simulink model "VU_motorSpdCtrl"  (Simulink 10.0)
settings: Solver=FixedStepDiscrete  StartTime=0.0  StopTime=inf  FixedStep=0.05  RelTol=1e-3  EnableMultiTasking=on
libraries: lego_nxt_lib x2
settings Model: Creator=jpeytonj  LastModifiedBy=bhisma
settings DataIOCC: LimitDataPoints=on  SignalLoggingSaveFormat=ModelDataLogs
settings OptimizationCC: ExpressionDepthLimit=2147483647
settings DebuggingCC: SolverPrmCheckMsg=warning  FcnCallInpInsideContextMsg=warning  StateNameClashWarn=warning
settings SFSimCC: SimParseCustomCode=off
settings RTWCC: Description=Lego NXT Real-Time Target  SystemTargetFile=lrt.tlc  GenCodeOnly=on  TemplateMakefile=lrt_ecrobot.tmf
settings STFCustomTargetCC: ModelReferenceCompliant=off  GeneratePreprocessorConditionals=Disable all  MatFileLogging=on  CPPClassGenCompliant=on  SystemTargetFile=lrt.tlc
settings GRTTargetCC: ModelReferenceCompliant=off  ParMdlRefBuildCompliant=off  CompOptLevelCompliant=off  ConcurrentExecutionCompliant=off  GeneratePreprocessorConditionals=Disable all  UseToolchainInfoCompliant=off  ExtModeMexFile=noextcomm
settings CustomProperty: DataType=RTWOptions_EnumType_C__LegoMindstorms_ECRobot_lrt_lrt_1codeGenType  Value=Integer-only
settings EnumStrPairs: String=Integer-only
settings ConfigComp: CovExternalEMLEnable=off

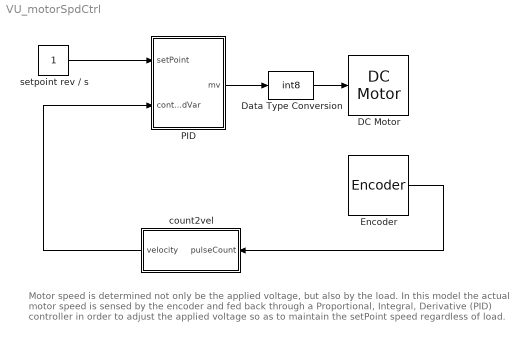
== system VU_motorSpdCtrl ==
  note: Motor speed is determined not only be the applied voltage, but also by the load.
      | In this model the actual motor speed is sensed by the encoder and fed back through
      | a Proportional, Integral, Derivative (PID) controller in order to adjust the applied voltage
      | so as to maintain the setPoint speed regardless of load.
  DC Motor : lego_nxt_lib/DC Motor  port=Port C  brake=Coast
  Data Type Conversion : DataTypeConversion  OutDataTypeStr=int8  SaturateOnIntegerOverflow=on
  Encoder : lego_nxt_lib/Encoder  port=Port C  st=0.05
  PID : Subsystem  mask{Kc=5.5, Ti=1.5, Td=0, mvMax=100, mvMin=-100}
      mask prompts: Kc "Proportional gain:"; Ti "Integral time:"; Td "Derivative time:"; mvMax "Max manipulated output Limit:"; mvMin "Min manipulated output Limit:"
  count2vel : Subsystem  mask(count2vel){gainFactor=1/0.05*1/360}
      mask prompts: gainFactor "Gain Factor:"
      mask help:
      | Use gainFactor to define units of the result:
      | If gainFactor=1, => units of velocity= (pulses/sample).
      | The encoders give 360 pulses / revolution of the output shaft
      |
      | Example:  To obtain velocity in rev/sec
      | velocity = (pulses/sample) * (samples/sec) * (rev/pulses) = rev/sec
      | Given a sample period T=0.1, and the known 360 pulses per rev...
      | => gainFactor = (1/0.1) * (1/360) = 1/36
      |
      | Not clear what happens when the pulse count overflows
  setpoint rev / s : Constant
  wires:
  PID/1(mv) -> Data Type Conversion/1
  setpoint rev / s/1 -> PID/1(setPoint)
  count2vel/1(velocity) -> PID/2(controlledVar)
  Data Type Conversion/1 -> DC Motor/1
  Encoder/1 -> count2vel/1(pulseCount)

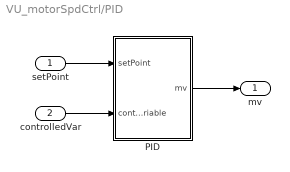
== system VU_motorSpdCtrl/PID ==
  setPoint : Inport
  controlledVar : Inport  Port=2
  PID : MATLAB Function  TreatAsAtomicUnit=on
  mv : Outport
  wires:
  setPoint/1 -> PID/1(setPoint)
  controlledVar/1 -> PID/2(contolledVariable)
  PID/1(mv) -> mv/1

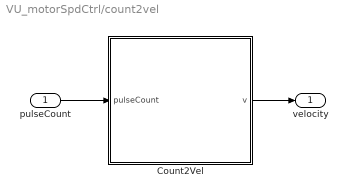
== system VU_motorSpdCtrl/count2vel ==
  pulseCount : Inport
  Count2Vel : MATLAB Function  TreatAsAtomicUnit=on
  velocity : Outport
  wires:
  pulseCount/1 -> Count2Vel/1(pulseCount)
  Count2Vel/1(v) -> velocity/1

== matlab function PID/PID ==
  data: setPoint input double; mv output double; contolledVariable input double; Kc parameter double; Ti parameter double; Td parameter double; mvMax parameter double; mvMin parameter double
function mv= PID (setPoint,contolledVariable,Kc,Ti,Td,mvMax,mvMin)

% PID uses the 'velocity algorithm' to drive the 
% 'controlledVariable' to follow the 'setPoint'  
% The manipulated variable is limited between 'mvMax' and 'mvMin'
% The controller proportional, integral and derivative gains are Kc, Ti, Td

% Date: 1 Oct 2010
% Author: JC Peyton Jones
% Villanova University

% Initialize persistent variables
persistent ekm1 ekm2 mvm1

if (isempty(ekm1)),
    ekm1= 0;        % e(k-1) is the error at time k-1
    ekm2= 0;        % e(k-2) is the error at time k-2
    mvm1= 0;        % mv(k-1) is the manipulated variable at k-1
end

% Compute the control action (the manipulated variable)
ek= setPoint - contolledVariable;
dm = Kc*(ek-ekm1 + (1/Ti)*ek + Td*(ek - 2*ekm1 + ekm2));
mv = mvm1 + dm;

% Limit the control action
if (mv > mvMax),
    mv = mvMax;
elseif (mv < mvMin),
    mv = mvMin;
end;

% Shift variables ready for next time
ekm2= ekm1;     % e(k-2)= e(k-1);
ekm1= ek;       % e(k-1)= e(k);
mvm1= mv;       % mv(k-1)= mv;

== matlab function count2vel/Count2Vel ==
  data: pulseCount input double; v output double; gainFactor parameter double
function v= velocity (pulseCount,gainFactor)

% Velocity computes the velocity in engineering units defined by gainFactor
% If gainFactor=1, => units are pulses/sample.  There are 360 pulses per rev
%
% Example:  To obtain velocity in rev/sec
% velocity = (pulses/sample) * (samples/sec) * (rev/pulses) = rev/sec
% Given a sample period T=0.1, and the known 360 pulses per rev...
% => gainFactor = (1/0.1) * (1/360) = 1/36
%
% Not clear what happens when the pulse count overflows


% Initialize persistent variables
persistent prevPulseCount

if (isempty(prevPulseCount)),
    prevPulseCount= int32(0); 
end

% Compute the velocity in units defined by gainFactor
v= double(pulseCount - prevPulseCount) * gainFactor;
prevPulseCount= pulseCount;
